simulink model "power_thermal"  (Simulink 6.0)
settings: Solver=ode23tb  StartTime=0.0  StopTime=0.5  MaxStep=50e-6  RelTol=1e-3
undefined symbols (not defined in the file or in its folder): D1, Delta
libraries: powerlib x21, powerlib_extras x1
settings Model: Creator=rchampag  LastModifiedBy=batserve  ExtModeTrigMode=oneshot  ExtModeArmWhenConnect=off  ExtModeAutoUpdateStatusClock=off
settings DataIOCC: LimitDataPoints=off  SaveOutput=off  SaveTime=off  TimeSaveName=t  SignalLoggingName=sigsOut
settings OptimizationCC: BlockReduction=off  BooleanDataType=off
settings DebuggingCC: CheckExecutionContextPreStartOutputMsg=on  CheckExecutionContextRuntimeOutputMsg=on  SolverPrmCheckMsg=none
settings HardwareCC: TargetUnknown=on

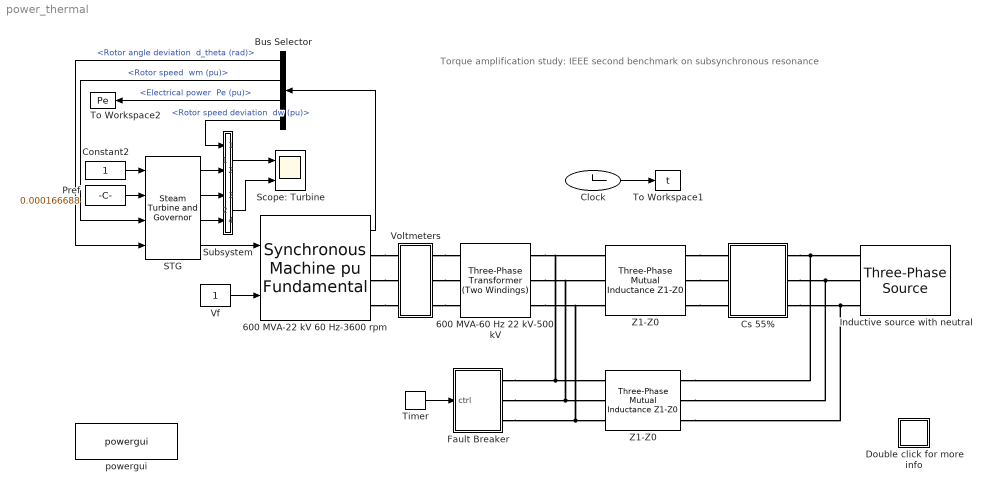
== system power_thermal ==
  note: Torque amplification study:
      | IEEE second benchmark on subsynchronous resonance
  600 MVA-22 kV 60 Hz-3600 rpm : powerlib/Machines/Synchronous Machine pu Fundamental  PresetModel=No  ShowDetailedParameters=on  RotorType=Round  NominalParameters="[ 600e6  22e3   60 ]"  Stator="[  0.0045  0.14  1.51  1.45 ]"  Field="[  0.00096  0.1186 ]"  Dampers2="[ 0.016  0.132  0.00898  0.411  0.0116  0.0738 ]"  Dampers1="[ 1.1685E-02  0.18167  1.9718E-02  038371 ]"  Mechanical="[ 0.87882   0.176*8   1 ]"  InitialConditions="[0  0   0 0 0   0 0 0   0]"  SetSaturation=off  Saturation=[0.6404,0.7127,0.8441,0.9214,0.9956,1.082,1.19,1.316,1.457;0.7,0.7698,0.8872,0.9466,0.9969,1.046,1.1,1.151,1.201]  Units=0  LoadFlowParameters=[1 100000 0 0]
      settings: AttributesFormatString=\n
  600 MVA-60 Hz 22 kV-500 kV : powerlib/Elements/Three-Phase Transformer (Two Windings)  NominalPower="[ 600e6   60 ]"  Winding1Connection=Delta (D1)  Winding1="[ 22e3  1e-6   0  ]"  Winding2Connection=Yg  Winding2="[ 500e3  0.0012   0.12 ]"  SetSaturation=off  Rm=500  Lm=500  Saturation="[ 0,0  ;  0.005,1.2  ;  1.0,1.4 ]"  Hysteresis=off  DataFile='hysteresis'  SetInitialFlux=off  InitialFluxes=[ 0.8 , -0.8 , 0.7 ]  Measurements=None  TransfoNumber=0
  Bus Selector : BusSelector  Orientation=left  DialogController=Simulink.DDGSource_Bus  OutputSignals="Mechanical.Rotor angle deviation  d_theta (rad),Mechanical.Rotor speed  wm (pu),Mechanical.Electrical power  Pe (pu),Mechanical.Rotor speed deviation  dw (pu)"
  Clock : Clock
      settings: Decimation=100
  Constant2 : Constant
  Cs 55% : Subsystem  Orientation=left
      mask Display: plot(0,0,100,100,[40,10],[50,50],[90,60],[50,50],[40,40],[20,80],[60,60],[20,80])
  Double click for more info : Subsystem
      mask Display: disp('?')
  Fault Breaker : Subsystem
  Inductive source with neutral : powerlib/Electrical Sources/Three-Phase Source  Orientation=left  Voltage=500e3  PhaseAngle=0  Frequency=60  InternalConnection=Yg  SpecifyImpedance=off  Resistance=3.5  Inductance=0.1989  ShortCircuitLevel=0  BaseVoltage=0  XRratio=0
  Pref : Constant  Value=0.000166688
  STG : powerlib/Machines/Steam Turbine and Governor  gentype=Tandem-compound (multi-mass)  reg1="[ 1  0.05    0 ]"  reg2="[ 0.001  0.15 ]"  reg3="[ -0.1  0.1  0.00016668  0.00016668*1.01 ]"  turb1="[ 0  10   3.3   0.5   ]"  turb2="[ 0.5   0.5   0  0 ]"  HA="[  1.5498   0.24894  0  0 ]"  KA="[  83.47  42.702  0  0 ]"  DA="[  0.3104  0.05  0  0 ]*8"  ini1=250.35/555  ini2=[0.000166688,-120.04]
  Scope: Turbine : Scope  NumInputPorts=2
      settings: TimeRange=0.5  YMin=-0.9~-70  YMax=0.6~130
  Subsystem : Subsystem
  Timer : powerlib_extras/Control  Blocks/Timer  t="[ 0.022289  0.022289+0.017 ]"  e=[ 1 0 ]
  To Workspace1 : ToWorkspace  VariableName=t  SaveFormat=Array
  To Workspace2 : ToWorkspace  VariableName=Pe  SaveFormat=Array
  Vf : Constant
  Voltmeters : Subsystem
  Z1-Z0 : powerlib/Elements/Three-Phase Mutual Inductance Z1-Z0  PhysicalDomain=powersysdomain  SubClassName=unknown  LeftPortType=p1  RightPortType=p1  LConnTagsString=a|b|c  RConnTagsString=A|B|C  PositiveSequence="[ 18.5  0.5305 ]"  ZeroSequence="[ 55.0  1.5915 ]"
  "Z1-Z0 " : powerlib/Elements/Three-Phase Mutual Inductance Z1-Z0  PhysicalDomain=powersysdomain  SubClassName=unknown  LeftPortType=p1  RightPortType=p1  LConnTagsString=a|b|c  RConnTagsString=A|B|C  PositiveSequence="[ 16.75  0.4901 ]"  ZeroSequence="[ 46.5  1.3926 ]"
  powergui : powerlib/powergui  Priority=2  Frange=logspace(0,3,50)  Ylog=off  Xlog=off  save=off  variable=ZData  ZoomFFT=on  StartTime=0.0  cycles=2  DisplayStyle=off  fundamental=60  FreqAxis=off  MaxFrequency=1000  frequencyindice=1  frequencyindicesteady=1  RmsSteady=1  display=off  Ts=0  methode=off  frequency=60  echomessages=off
  wires:
  Constant2/1 -> STG/1
  Bus Selector/1 -> STG/4  "<Rotor angle deviation  d_theta (rad)>"
  Pref/1 -> STG/2
  STG/1 -> Subsystem/2(In2)
  Subsystem/2(Out2) -> Scope: Turbine/2
  Bus Selector/2 -> STG/3  "<Rotor speed  wm (pu)>"
  Bus Selector/4 -> Subsystem/1(In1)  "<Rotor speed deviation  dw (pu)>"
  Subsystem/1(Out1) -> Scope: Turbine/1
  STG/2 -> Subsystem/3(In3)
  Bus Selector/3 -> To Workspace2/1  "<Electrical power  Pe (pu)>"
  Timer/1 -> Fault Breaker/1(ctrl)
  Clock/1 -> To Workspace1/1
  STG/3 -> Subsystem/4(In4)
  Vf/1 -> 600 MVA-22 kV 60 Hz-3600 rpm/2
  600 MVA-22 kV 60 Hz-3600 rpm/1 -> Bus Selector/1
  STG/4 -> 600 MVA-22 kV 60 Hz-3600 rpm/1
  connections:
  600 MVA-22 kV 60 Hz-3600 rpm/RConn1 -- Voltmeters/LConn1
  Voltmeters/RConn1 -- 600 MVA-60 Hz 22 kV-500 kV/LConn1
  600 MVA-22 kV 60 Hz-3600 rpm/RConn2 -- Voltmeters/LConn2
  600 MVA-22 kV 60 Hz-3600 rpm/RConn3 -- Voltmeters/LConn3
  Voltmeters/RConn2 -- 600 MVA-60 Hz 22 kV-500 kV/LConn2
  Voltmeters/RConn3 -- 600 MVA-60 Hz 22 kV-500 kV/LConn3
  Fault Breaker/RConn2 -- 600 MVA-60 Hz 22 kV-500 kV/RConn2 -- Z1-Z0/LConn2 -- "Z1-Z0 "/LConn2
  600 MVA-60 Hz 22 kV-500 kV/RConn1 -- Z1-Z0/LConn1 -- "Z1-Z0 "/LConn1 -- Fault Breaker/RConn1
  600 MVA-60 Hz 22 kV-500 kV/RConn3 -- Z1-Z0/LConn3 -- "Z1-Z0 "/LConn3 -- Fault Breaker/RConn3
  Z1-Z0/RConn2 -- Cs 55%/RConn2
  Z1-Z0/RConn1 -- Cs 55%/RConn1
  Z1-Z0/RConn3 -- Cs 55%/RConn3
  Cs 55%/LConn2 -- Inductive source with neutral/RConn2 -- "Z1-Z0 "/RConn2
  Cs 55%/LConn3 -- Inductive source with neutral/RConn3 -- "Z1-Z0 "/RConn3
  Cs 55%/LConn1 -- Inductive source with neutral/RConn1 -- "Z1-Z0 "/RConn1

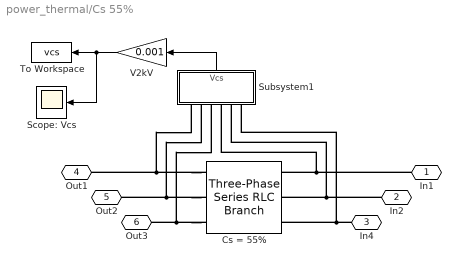
== system power_thermal/Cs 55% ==
  Cs = 55% : powerlib/Elements/Three-Phase Series RLC Branch  Orientation=left  PhysicalDomain=powersysdomain  SubClassName=unknown  LeftPortType=p1  RightPortType=p1  LConnTagsString=A|B|C  RConnTagsString=A|B|C  Resistance=0  Inductance=0  Capacitance=1/(0.55*0.5305*(120*pi)^2)  Measurements=None
  Scope: Vcs : Scope
      settings: YMin=-500  YMax=500
  Subsystem1 : Subsystem  Orientation=up
  To Workspace : ToWorkspace  VariableName=vcs  SaveFormat=Array
  V2kV : Gain  Orientation=left  Gain=0.001  SaturateOnIntegerOverflow=on
  In1 : PMIOPort  Orientation=left  Port=1  Side=Left
  In2 : PMIOPort  Orientation=left  Port=2  Side=Left
  In4 : PMIOPort  Orientation=left  Port=3  Side=Left
  Out1 : PMIOPort  Port=4  Side=Right
  Out2 : PMIOPort  Port=5  Side=Right
  Out3 : PMIOPort  Port=6  Side=Right
  wires:
  Subsystem1/1(Vcs) -> V2kV/1
  V2kV/1 -> To Workspace/1, Scope: Vcs/1
  connections:
  Cs = 55%/RConn1 -- Subsystem1/LConn1 -- Out1/RConn1
  Cs = 55%/RConn2 -- Subsystem1/LConn2 -- Out2/RConn1
  Cs = 55%/RConn3 -- Subsystem1/LConn3 -- Out3/RConn1
  In2/RConn1 -- Cs = 55%/LConn2 -- Subsystem1/LConn5
  In4/RConn1 -- Cs = 55%/LConn3 -- Subsystem1/LConn6
  In1/RConn1 -- Cs = 55%/LConn1 -- Subsystem1/LConn4

== system power_thermal/Double click for more info ==
  note: This system is an IEEE benchmark [1] used to study subsynchronous resonance and particularly torque amplification
      | after a fault on a series-compensated power system. It consists in a single generator (600 MVA/22kV/60 Hz/3600 rpm)
      | connected to an infinite bus via two transmission lines, one of which is series-compensated. The subsynchronous
      | mode introduced by the compensation capacitor after a fault has been applied and cleared excites the oscillatory
      | torsional modes of the multi-mass shaft and the torque amplification phenomenon can be observed.
  note: This demonstration illustrates subsynchronous resonance (SSR)
      | using the Steam Turbine and Governor on a series-compensated network
  note: Circuit Description
  note: Demonstration
  note: Reference
  note: [1] IEEE Subsynchronous resonance working group, "Second benchmark model for computer simulation of subsynchronous
      |      resonance," IEEE Transactions on Power Apparatus and Systems, vol. PAS-104, no. 5, 1985, pp. 1057-1066.
  note: Louis-A. Dessaint and R. Champagne (Ecole de Technologie Superieure, Montreal)
  note: Open the Scope connected to the STG model. Run the simulation by selecting Start from the Simulation menu.
      | Observe the speed deviations on the top axis of the Scope and the torques transmitted between the shaft's
      | masses on the bottom axis. A peak torque of over 4 pu is observed between masses 1 and 2. The frequency
      | of the oscillations oberved in the torques and speed deviations is about 27 Hz. Excellent aggreement between
      | peak values observed here and those given in [1] is obtained.
  note: 1
  note: Open the synchronous machine (SM) block menu and observe that the machine intial conditions (last line)  are set to zero.
      | Start Simulation. As the SM initial conditions are not properly set you will observe that simulation does not start in steady state.
      | Stop the simulation.
  note: 2
  note: In order to start the simulation in steady-state you must initialize the synchronous machine for the desired load flow.
      | Open the  POWERGUI and select "Load Flow & Machine initialization" . The machine "Bus type" should be already initialized as "PV generator",
      | indicating that  the load flow will be performed with the machine controlling its active power and terminal voltage.
      | Specify the desired values by entering the following parameters:
  note: Load Flow: U AB (Vrms) = 22000 , P (wattts) =100e3
  note: Then press the "Update Load Flow" button.
      |
      | Once the load flow is solved the phasors of AB and BC machine voltages and currents flowing in phases A and B are updated.
      | The SM reactive power,  mechanical power and  field voltage are displayed : Q = 1.30 Mvar, Pmec = 100 kW (0.0001667 pu), field voltage Ef = 1.0036 pu;
      | If you open the SM block menu you will observe that the initial conditions have been updated.
  note: In order to start the simulation in steady state with the STG connected, this Simulink block must also be initialized according to the values
      | calculated by the load flow. This initialization is automatically performed when you execute the Load Flow, as long as you connect  at
      | the Pm and Vf inputs of the machine either Constant blocks or regulation blocks from the machine library (HTG, STG, or Excitation System).
      | Open the STG block menu and notice that the initial mechanical power and generator rotor angle have been automatically set to
      | Pm0=0.0001667 pu  (100.01 kW) and th0 = -120.04 degrees by the Load Flow. The Vf constant block connected at the Vf excitation input of the synchronous
      | machine has been automaticlly set to 1.00358 pu by the Load Flow. The Pref constant block connected at the Pref input of the STG block
      | has also been updated.
  note: 3
  note: 4

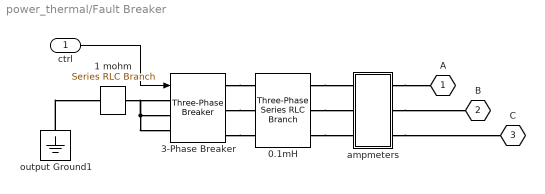
== system power_thermal/Fault Breaker ==
  ctrl : Inport  Port=1  LatchInput=off
  0.1mH : powerlib/Elements/Three-Phase Series RLC Branch  PhysicalDomain=powersysdomain  SubClassName=unknown  LeftPortType=p1  RightPortType=p1  LConnTagsString=A|B|C  RConnTagsString=A|B|C  Resistance=0  Inductance=0.1e-3  Capacitance=inf  Measurements=None
  1 mohm : powerlib/Elements/Series RLC Branch  PhysicalDomain=powersysdomain  SubClassName=unknown  LeftPortType=p1  RightPortType=p1  LConnTagsString=__new0  RConnTagsString=__new0  Resistance=0.001  Inductance=0  Capacitance=inf  Measurements=None
  3-Phase Breaker : powerlib/Elements/Three-Phase Breaker  InitialState=open  SwitchA=on  SwitchB=on  SwitchC=on  SwitchTimes="[4/60  10/60]"  External=on  BreakerResistance=0.001  SnubberResistance=1e6  SnubberCapacitance=inf  Measurements=None
      settings: AttributesFormatString=\n
  ampmeters : Subsystem
  output Ground1 : powerlib/Elements/Ground  Orientation=down  PhysicalDomain=powersysdomain  SubClassName=unknown  LeftPortType=p1  RightPortType=p1  LConnTagsString=a
  A : PMIOPort  Orientation=left  Port=1  Side=Right
  B : PMIOPort  Orientation=left  Port=2  Side=Right
  C : PMIOPort  Orientation=left  Port=3  Side=Right
  wires:
  ctrl/1 -> 3-Phase Breaker/1
  connections:
  3-Phase Breaker/RConn1 -- 0.1mH/LConn1
  3-Phase Breaker/RConn2 -- 0.1mH/LConn2
  3-Phase Breaker/RConn3 -- 0.1mH/LConn3
  0.1mH/RConn3 -- ampmeters/LConn3
  0.1mH/RConn2 -- ampmeters/LConn2
  0.1mH/RConn1 -- ampmeters/LConn1
  output Ground1/LConn1 -- 1 mohm/LConn1
  1 mohm/RConn1 -- 3-Phase Breaker/LConn1 -- 3-Phase Breaker/LConn2 -- 3-Phase Breaker/LConn3
  ampmeters/RConn1 -- A/RConn1
  ampmeters/RConn2 -- B/RConn1
  ampmeters/RConn3 -- C/RConn1

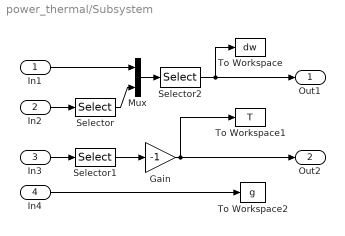
== system power_thermal/Subsystem ==
  In1 : Inport  Port=1  LatchInput=off
  In2 : Inport  Port=2  LatchInput=off
  In3 : Inport  Port=3  LatchInput=off
  In4 : Inport  Port=4  LatchInput=off
  Gain : Gain  Gain=-1  SaturateOnIntegerOverflow=on
  Mux : Mux  Inputs=2
  Selector : Selector  Elements=[3 4]  InputPortWidth=4
  Selector1 : Selector  Elements=[3 4]  InputPortWidth=4
  Selector2 : Selector  Elements=[2 3 1]  InputPortWidth=3
  To Workspace : ToWorkspace  VariableName=dw  SaveFormat=Array
  To Workspace1 : ToWorkspace  VariableName=T  SaveFormat=Array
  To Workspace2 : ToWorkspace  VariableName=g  SaveFormat=Array
  Out1 : Outport
  Out2 : Outport  Port=2
  wires:
  Selector/1 -> Mux/2
  Mux/1 -> Selector2/1
  In1/1 -> Mux/1
  In2/1 -> Selector/1
  In3/1 -> Selector1/1
  Selector2/1 -> Out1/1, To Workspace/1
  In4/1 -> To Workspace2/1
  Selector1/1 -> Gain/1
  Gain/1 -> To Workspace1/1, Out2/1

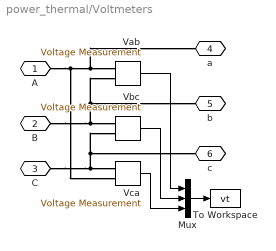
== system power_thermal/Voltmeters ==
  Mux : Mux  Inputs=3
  To Workspace : ToWorkspace  VariableName=vt  SaveFormat=Array
  Vab : powerlib/Measurements/Voltage Measurement  Tag=PoWeRsYsTeMmEaSuReMeNt  PhasorSimulation=off  OutputType=Magnitude  PSBequivalent=0
  Vbc : powerlib/Measurements/Voltage Measurement  Tag=PoWeRsYsTeMmEaSuReMeNt  PhasorSimulation=off  OutputType=Magnitude  PSBequivalent=0
  Vca : powerlib/Measurements/Voltage Measurement  Tag=PoWeRsYsTeMmEaSuReMeNt  PhasorSimulation=off  OutputType=Magnitude  PSBequivalent=0
  A : PMIOPort  Port=1  Side=Left
  B : PMIOPort  Port=2  Side=Left
  C : PMIOPort  Port=3  Side=Left
  a : PMIOPort  Orientation=left  Port=4  Side=Right
  b : PMIOPort  Orientation=left  Port=5  Side=Right
  c : PMIOPort  Orientation=left  Port=6  Side=Right
  wires:
  Mux/1 -> To Workspace/1
  Vca/1 -> Mux/3
  Vbc/1 -> Mux/2
  Vab/1 -> Mux/1
  connections:
  B/RConn1 -- Vbc/LConn1 -- Vab/LConn2 -- b/RConn1
  C/RConn1 -- Vca/LConn1 -- Vbc/LConn2 -- c/RConn1
  A/RConn1 -- Vab/LConn1 -- a/RConn1 -- Vca/LConn2

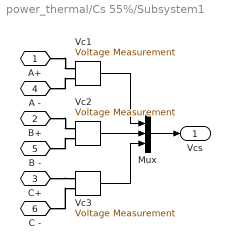
== system power_thermal/Cs 55%/Subsystem1 ==
  Mux : Mux  Inputs=3
  Vc1 : powerlib/Measurements/Voltage Measurement  Tag=PoWeRsYsTeMmEaSuReMeNt  PhasorSimulation=off  OutputType=Magnitude  PSBequivalent=0
  Vc2 : powerlib/Measurements/Voltage Measurement  Tag=PoWeRsYsTeMmEaSuReMeNt  PhasorSimulation=off  OutputType=Magnitude  PSBequivalent=0
  Vc3 : powerlib/Measurements/Voltage Measurement  Tag=PoWeRsYsTeMmEaSuReMeNt  PhasorSimulation=off  OutputType=Magnitude  PSBequivalent=0
  A+ : PMIOPort  Port=1  Side=Left
  B+ : PMIOPort  Port=2  Side=Left
  C+ : PMIOPort  Port=3  Side=Left
  A - : PMIOPort  Port=4  Side=Left
  B - : PMIOPort  Port=5  Side=Left
  C - : PMIOPort  Port=6  Side=Left
  Vcs : Outport
  wires:
  Mux/1 -> Vcs/1
  Vc1/1 -> Mux/1
  Vc2/1 -> Mux/2
  Vc3/1 -> Mux/3
  connections:
  C+/RConn1 -- Vc3/LConn1
  C -/RConn1 -- Vc3/LConn2
  B+/RConn1 -- Vc2/LConn1
  B -/RConn1 -- Vc2/LConn2
  A+/RConn1 -- Vc1/LConn1
  A -/RConn1 -- Vc1/LConn2

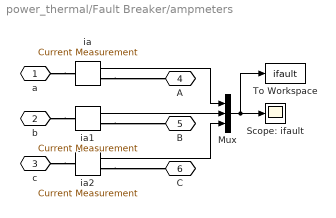
== system power_thermal/Fault Breaker/ampmeters ==
  Mux : Mux  Inputs=3
  Scope: ifault : Scope
      settings: YMin=-9000  YMax=9000
  To Workspace : ToWorkspace  VariableName=ifault  SaveFormat=Array
  ia : powerlib/Measurements/Current Measurement  Tag=PoWeRsYsTeMmEaSuReMeNt  PhasorSimulation=off  OutputType=Magnitude  PSBequivalent=0
  ia1 : powerlib/Measurements/Current Measurement  Tag=PoWeRsYsTeMmEaSuReMeNt  PhasorSimulation=off  OutputType=Magnitude  PSBequivalent=0
  ia2 : powerlib/Measurements/Current Measurement  Tag=PoWeRsYsTeMmEaSuReMeNt  PhasorSimulation=off  OutputType=Magnitude  PSBequivalent=0
  a : PMIOPort  Port=1  Side=Left
  b : PMIOPort  Port=2  Side=Left
  c : PMIOPort  Port=3  Side=Left
  A : PMIOPort  Orientation=left  Port=4  Side=Right
  B : PMIOPort  Orientation=left  Port=5  Side=Right
  C : PMIOPort  Orientation=left  Port=6  Side=Right
  wires:
  Mux/1 -> Scope: ifault/1, To Workspace/1
  ia/1 -> Mux/1
  ia1/1 -> Mux/2
  ia2/1 -> Mux/3
  connections:
  a/RConn1 -- ia/LConn1
  b/RConn1 -- ia1/LConn1
  c/RConn1 -- ia2/LConn1
  ia/RConn1 -- A/RConn1
  ia1/RConn1 -- B/RConn1
  ia2/RConn1 -- C/RConn1
